simulink model "FFT_32_point_fi_RTL_Implementation"  (R2021a)
settings: Solver=VariableStepAuto  StartTime=0.0  StopTime=0.00001  RelTol=1e-3
undefined symbols (not defined in the file): Input, W16, W2, W32, W4, W8
settings Model: Creator=bahyy  LastModifiedBy=bahyy

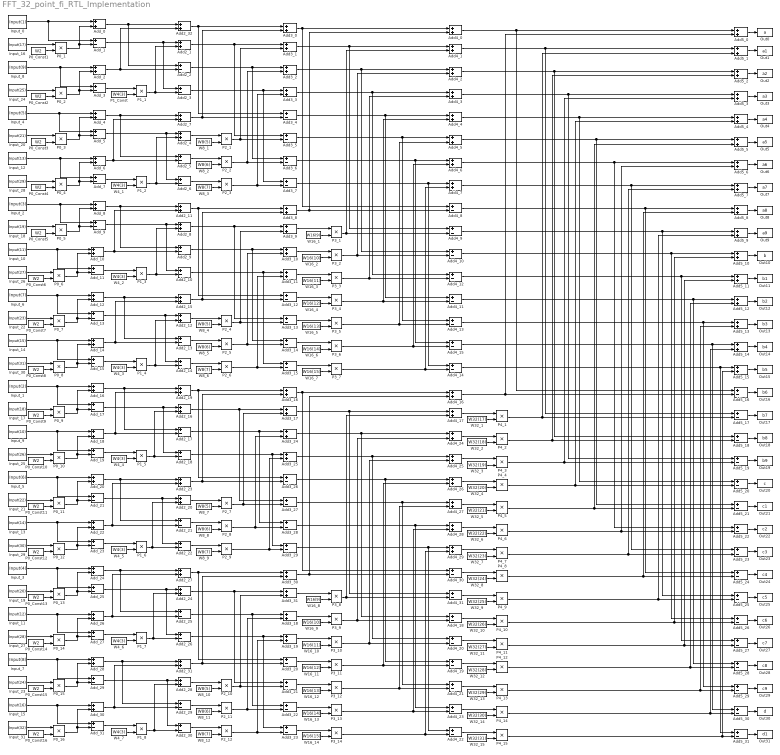
== system FFT_32_point_fi_RTL_Implementation ==
  Add2_{1,4,8,12,16,20,24,28} (8 alike) : Sum  InputSameDT=on  AccumDataTypeStr=fixdt(1,N_bits,W_bits-1)  OutDataTypeStr=fixdt(1,N_bits,W_bits-1)
  Add2_{2..3,5..6,9..10,13..14,17..18,21..22,25..26,29..30} (16 alike) : Sum  Inputs=+-  AccumDataTypeStr=fixdt(1,N_bits,W_bits-1)  OutDataTypeStr=fixdt(1,N_bits,W_bits-1)
  Add2_{7,11,15,19,23,27,31..32} (8 alike) : Sum  AccumDataTypeStr=fixdt(1,N_bits,W_bits-1)  OutDataTypeStr=fixdt(1,N_bits,W_bits-1)
  Add3_{0..3,8..11,16..19,24..25,30..31} (16 alike) : Sum  AccumDataTypeStr=fixdt(1,N_bits,W_bits-1)  OutDataTypeStr=fixdt(1,N_bits,W_bits-1)
  Add3_{4..7,12..15,20..23,26..29} (16 alike) : Sum  Inputs=+-  AccumDataTypeStr=fixdt(1,N_bits,W_bits-1)  OutDataTypeStr=fixdt(1,N_bits,W_bits-1)
  Add4_{0..7,16..17,24..29} (16 alike) : Sum  AccumDataTypeStr=fixdt(1,N_bits,W_bits-1)  OutDataTypeStr=fixdt(1,N_bits,W_bits-1)
  Add4_{8..15,18..23,30..31} (16 alike) : Sum  Inputs=+-  AccumDataTypeStr=fixdt(1,N_bits,W_bits-1)  OutDataTypeStr=fixdt(1,N_bits,W_bits-1)
  Add5_{0..15} (16 alike) : Sum  AccumDataTypeStr=fixdt(1,N_bits,W_bits-1)  OutDataTypeStr=fixdt(1,N_bits,W_bits-1)
  Add5_{16..31} (16 alike) : Sum  Inputs=+-  AccumDataTypeStr=fixdt(1,N_bits,W_bits-1)  OutDataTypeStr=fixdt(1,N_bits,W_bits-1)
  Add_{0,2,4,6,8,10,12,14,16,18,20,22,24,26,28,30} (16 alike) : Sum  AccumDataTypeStr=fixdt(1,N_bits,W_bits-1)  OutDataTypeStr=fixdt(1,N_bits,W_bits-1)
  Add_{1,3,5,7,9,11,13,15,17,19,21,23,25,27,29,31} (16 alike) : Sum  Inputs=+-  AccumDataTypeStr=fixdt(1,N_bits,W_bits-1)  OutDataTypeStr=fixdt(1,N_bits,W_bits-1)
  Input_0 : Constant  Value=Input(1)
  Input_1 : Constant  Value=Input(2)
  Input_10 : Constant  Value=Input(11)
  Input_11 : Constant  Value=Input(12)
  Input_12 : Constant  Value=Input(13)
  Input_13 : Constant  Value=Input(14)
  Input_14 : Constant  Value=Input(15)
  Input_15 : Constant  Value=Input(16)
  Input_16 : Constant  Value=Input(17)
  Input_17 : Constant  Value=Input(18)
  Input_18 : Constant  Value=Input(19)
  Input_19 : Constant  Value=Input(20)
  Input_2 : Constant  Value=Input(3)
  Input_20 : Constant  Value=Input(21)
  Input_21 : Constant  Value=Input(22)
  Input_22 : Constant  Value=Input(23)
  Input_23 : Constant  Value=Input(24)
  Input_24 : Constant  Value=Input(25)
  Input_25 : Constant  Value=Input(26)
  Input_26 : Constant  Value=Input(27)
  Input_27 : Constant  Value=Input(28)
  Input_28 : Constant  Value=Input(29)
  Input_29 : Constant  Value=Input(30)
  Input_3 : Constant  Value=Input(4)
  Input_30 : Constant  Value=Input(31)
  Input_31 : Constant  Value=Input(32)
  Input_4 : Constant  Value=Input(5)
  Input_5 : Constant  Value=Input(6)
  Input_6 : Constant  Value=Input(7)
  Input_7 : Constant  Value=Input(8)
  Input_8 : Constant  Value=Input(9)
  Input_9 : Constant  Value=Input(10)
  Out0 : ToWorkspace  VariableName=a  SampleTime=1
      settings: MaxDataPoints=1  Save2DSignal=2-D array (concatenate along first dimension)
  Out1 : ToWorkspace  VariableName=a1  SampleTime=1
      settings: MaxDataPoints=1  Save2DSignal=2-D array (concatenate along first dimension)
  Out10 : ToWorkspace  VariableName=b  SampleTime=1
      settings: MaxDataPoints=1  Save2DSignal=2-D array (concatenate along first dimension)
  Out11 : ToWorkspace  VariableName=b1  SampleTime=1
      settings: MaxDataPoints=1  Save2DSignal=2-D array (concatenate along first dimension)
  Out12 : ToWorkspace  VariableName=b2  SampleTime=1
      settings: MaxDataPoints=1  Save2DSignal=2-D array (concatenate along first dimension)
  Out13 : ToWorkspace  VariableName=b3  SampleTime=1
      settings: MaxDataPoints=1  Save2DSignal=2-D array (concatenate along first dimension)
  Out14 : ToWorkspace  VariableName=b4  SampleTime=1
      settings: MaxDataPoints=1  Save2DSignal=2-D array (concatenate along first dimension)
  Out15 : ToWorkspace  VariableName=b5  SampleTime=1
      settings: MaxDataPoints=1  Save2DSignal=2-D array (concatenate along first dimension)
  Out16 : ToWorkspace  VariableName=b6  SampleTime=1
      settings: MaxDataPoints=1  Save2DSignal=2-D array (concatenate along first dimension)
  Out17 : ToWorkspace  VariableName=b7  SampleTime=1
      settings: MaxDataPoints=1  Save2DSignal=2-D array (concatenate along first dimension)
  Out18 : ToWorkspace  VariableName=b8  SampleTime=1
      settings: MaxDataPoints=1  Save2DSignal=2-D array (concatenate along first dimension)
  Out19 : ToWorkspace  VariableName=b9  SampleTime=1
      settings: MaxDataPoints=1  Save2DSignal=2-D array (concatenate along first dimension)
  Out2 : ToWorkspace  VariableName=a2  SampleTime=1
      settings: MaxDataPoints=1  Save2DSignal=2-D array (concatenate along first dimension)
  Out20 : ToWorkspace  VariableName=c  SampleTime=1
      settings: MaxDataPoints=1  Save2DSignal=2-D array (concatenate along first dimension)
  Out21 : ToWorkspace  VariableName=c1  SampleTime=1
      settings: MaxDataPoints=1  Save2DSignal=2-D array (concatenate along first dimension)
  Out22 : ToWorkspace  VariableName=c2  SampleTime=1
      settings: MaxDataPoints=1  Save2DSignal=2-D array (concatenate along first dimension)
  Out23 : ToWorkspace  VariableName=c3  SampleTime=1
      settings: MaxDataPoints=1  Save2DSignal=2-D array (concatenate along first dimension)
  Out24 : ToWorkspace  VariableName=c4  SampleTime=1
      settings: MaxDataPoints=1  Save2DSignal=2-D array (concatenate along first dimension)
  Out25 : ToWorkspace  VariableName=c5  SampleTime=1
      settings: MaxDataPoints=1  Save2DSignal=2-D array (concatenate along first dimension)
  Out26 : ToWorkspace  VariableName=c6  SampleTime=1
      settings: MaxDataPoints=1  Save2DSignal=2-D array (concatenate along first dimension)
  Out27 : ToWorkspace  VariableName=c7  SampleTime=1
      settings: MaxDataPoints=1  Save2DSignal=2-D array (concatenate along first dimension)
  Out28 : ToWorkspace  VariableName=c8  SampleTime=1
      settings: MaxDataPoints=1  Save2DSignal=2-D array (concatenate along first dimension)
  Out29 : ToWorkspace  VariableName=c9  SampleTime=1
      settings: MaxDataPoints=1  Save2DSignal=2-D array (concatenate along first dimension)
  Out3 : ToWorkspace  VariableName=a3  SampleTime=1
      settings: MaxDataPoints=1  Save2DSignal=2-D array (concatenate along first dimension)
  Out30 : ToWorkspace  VariableName=d  SampleTime=1
      settings: MaxDataPoints=1  Save2DSignal=2-D array (concatenate along first dimension)
  Out31 : ToWorkspace  VariableName=d1  SampleTime=1
      settings: MaxDataPoints=1  Save2DSignal=2-D array (concatenate along first dimension)
  Out4 : ToWorkspace  VariableName=a4  SampleTime=1
      settings: MaxDataPoints=1  Save2DSignal=2-D array (concatenate along first dimension)
  Out5 : ToWorkspace  VariableName=a5  SampleTime=1
      settings: MaxDataPoints=1  Save2DSignal=2-D array (concatenate along first dimension)
  Out6 : ToWorkspace  VariableName=a6  SampleTime=1
      settings: MaxDataPoints=1  Save2DSignal=2-D array (concatenate along first dimension)
  Out7 : ToWorkspace  VariableName=a7  SampleTime=1
      settings: MaxDataPoints=1  Save2DSignal=2-D array (concatenate along first dimension)
  Out8 : ToWorkspace  VariableName=a8  SampleTime=1
      settings: MaxDataPoints=1  Save2DSignal=2-D array (concatenate along first dimension)
  Out9 : ToWorkspace  VariableName=a9  SampleTime=1
      settings: MaxDataPoints=1  Save2DSignal=2-D array (concatenate along first dimension)
  P0_{1..16} (16 alike) : Product  OutDataTypeStr=fixdt(1,N_bits,W_bits-1)
  P0_Const{1..16} (16 alike) : Constant  Value=W2
  P1_{1..8} (8 alike) : Product  OutDataTypeStr=fixdt(1,N_bits,W_bits-1)
  P1_Const : Constant  Value=W4(3)
  P2_{1..12} (12 alike) : Product  OutDataTypeStr=fixdt(1,N_bits,W_bits-1)
  P3_{1..14} (14 alike) : Product  OutDataTypeStr=fixdt(1,N_bits,W_bits-1)
  P4_{1..15} (15 alike) : Product  OutDataTypeStr=fixdt(1,N_bits,W_bits-1)
  W16_1 : Constant  Value=W16(9)
  W16_10 : Constant  Value=W16(11)
  W16_11 : Constant  Value=W16(12)
  W16_12 : Constant  Value=W16(13)
  W16_13 : Constant  Value=W16(14)
  W16_14 : Constant  Value=W16(15)
  W16_2 : Constant  Value=W16(10)
  W16_3 : Constant  Value=W16(11)
  W16_4 : Constant  Value=W16(12)
  W16_5 : Constant  Value=W16(13)
  W16_6 : Constant  Value=W16(14)
  W16_7 : Constant  Value=W16(15)
  W16_8 : Constant  Value=W16(9)
  W16_9 : Constant  Value=W16(10)
  W32_1 : Constant  Value=W32(17)
  W32_10 : Constant  Value=W32(26)
  W32_11 : Constant  Value=W32(27)
  W32_12 : Constant  Value=W32(28)
  W32_13 : Constant  Value=W32(29)
  W32_14 : Constant  Value=W32(30)
  W32_15 : Constant  Value=W32(31)
  W32_2 : Constant  Value=W32(18)
  W32_3 : Constant  Value=W32(19)
  W32_4 : Constant  Value=W32(20)
  W32_5 : Constant  Value=W32(21)
  W32_6 : Constant  Value=W32(22)
  W32_7 : Constant  Value=W32(23)
  W32_8 : Constant  Value=W32(24)
  W32_9 : Constant  Value=W32(25)
  W4_{1..7} (7 alike) : Constant  Value=W4(3)
  W8_{1,4,7,10} (4 alike) : Constant  Value=W8(5)
  W8_{2,5,8,11} (4 alike) : Constant  Value=W8(6)
  W8_{3,6,9,12} (4 alike) : Constant  Value=W8(7)
  wires:
  Add5_0/1 -> Out0/1
  Add5_6/1 -> Out6/1
  P2_5/1 -> Add3_14/2, Add3_10/2
  Input_4/1 -> Add_5/1, Add_4/1
  P2_1/1 -> Add3_1/2, Add3_5/2
  Add3_6/1 -> Add4_15/1, Add4_6/1
  P3_10/1 -> Add4_20/2, Add4_25/2
  Add5_18/1 -> Out18/1
  W4_1/1 -> P1_2/2
  Add_28/1 -> Add2_29/1, Add2_31/1
  Add2_23/1 -> Add3_26/2, Add3_16/2
  Add5_20/1 -> Out20/1
  Add3_3/1 -> Add4_12/1, Add4_3/1
  Add_14/1 -> Add2_15/2, Add2_13/2
  Add4_17/1 -> P4_1/1
  Add4_13/1 -> Add5_29/1, Add5_13/1
  P4_12/1 -> Add5_28/2, Add5_12/2
  Add_16/1 -> Add2_19/1, Add2_17/1
  P2_11/1 -> Add3_18/2, Add3_22/2
  Add4_7/1 -> Add5_23/1, Add5_7/1
  P2_8/1 -> Add3_28/2, Add3_24/2
  P3_9/1 -> Add4_18/2, Add4_24/2
  W16_6/1 -> P3_6/2
  Add_17/1 -> Add2_18/1, Add2_16/1
  Add4_11/1 -> Add5_28/1, Add5_12/1
  P4_8/1 -> Add5_24/2, Add5_8/2
  W16_4/1 -> P3_4/2
  Add3_11/1 -> P3_3/1
  P4_15/1 -> Add5_31/2, Add5_15/2
  Add5_22/1 -> Out22/1
  Add_23/1 -> P1_6/1
  W16_7/1 -> P3_7/2
  W16_12/1 -> P3_12/2
  Add4_2/1 -> Add5_18/1, Add5_2/1
  Add_31/1 -> P1_8/1
  W32_4/1 -> P4_4/2
  Add_27/1 -> P1_7/1
  P3_4/1 -> Add4_11/2, Add4_4/2
  W16_1/1 -> P3_1/2
  P1_7/1 -> Add2_24/2, Add2_26/2
  W8_5/1 -> P2_5/2
  Add_10/1 -> Add2_11/2, Add2_9/2
  W4_4/1 -> P1_5/2
  Add5_23/1 -> Out23/1
  P3_5/1 -> Add4_13/2, Add4_5/2
  Add_3/1 -> P1_1/1
  P4_5/1 -> Add5_21/2, Add5_5/2
  P1_Const/1 -> P1_1/2
  W32_14/1 -> P4_14/2
  Add5_11/1 -> Out11/1
  Add3_20/1 -> P3_11/1
  Add3_1/1 -> Add4_9/1, Add4_1/1
  Add3_0/1 -> Add4_8/1, Add4_0/1
  Add2_4/1 -> P2_1/1
  Add_24/1 -> Add2_25/1, Add2_27/1
  Add3_30/1 -> Add4_16/2, Add4_30/2
  W4_3/1 -> P1_4/2
  Add_4/1 -> Add2_7/1, Add2_5/1
  Add5_1/1 -> Out1/1
  Add2_8/1 -> Add3_13/1, Add3_9/1
  P4_9/1 -> Add5_25/2, Add5_9/2
  W16_2/1 -> P3_2/2
  P1_4/1 -> Add2_14/2, Add2_12/2
  Add_8/1 -> Add2_9/1, Add2_11/1
  Add5_14/1 -> Out14/1
  Add3_19/1 -> P3_10/1
  Add_9/1 -> Add2_10/1, Add2_8/1
  Add2_1/1 -> Add3_5/1, Add3_1/1
  Add_6/1 -> Add2_7/2, Add2_5/2
  Add4_4/1 -> Add5_20/1, Add5_4/1
  Add_1/1 -> Add2_3/1, Add2_1/1
  Add2_10/1 -> Add3_15/1, Add3_11/1
  W4_2/1 -> P1_3/2
  Add2_27/1 -> Add3_20/1, Add3_30/1
  W32_9/1 -> P4_9/2
  Add5_27/1 -> Out27/1
  W16_14/1 -> P3_14/2
  Add5_3/1 -> Out3/1
  Add5_15/1 -> Out15/1
  P2_2/1 -> Add3_6/2, Add3_2/2
  W4_7/1 -> P1_8/2
  Add_30/1 -> Add2_29/2, Add2_31/2
  P4_7/1 -> Add5_23/2, Add5_7/2
  P1_8/1 -> Add2_30/2, Add2_28/2
  P3_7/1 -> Add4_14/2, Add4_7/2
  P4_1/1 -> Add5_17/2, Add5_1/2
  W16_9/1 -> P3_9/2
  Add4_26/1 -> P4_4/1
  W32_1/1 -> P4_1/2
  Add_2/1 -> Add2_32/2, Add2_2/2
  Add_0/1 -> Add2_32/1, Add2_2/1
  Add5_26/1 -> Out26/1
  P2_7/1 -> Add3_17/2, Add3_27/2
  Add5_29/1 -> Out29/1
  P3_8/1 -> Add4_17/2, Add4_31/2
  Add_25/1 -> Add2_24/1, Add2_26/1
  Add2_22/1 -> P2_9/1
  Add3_16/1 -> Add4_16/1, Add4_30/1
  P3_12/1 -> Add4_27/2, Add4_21/2
  Add2_17/1 -> Add3_28/1, Add3_24/1
  P1_6/1 -> Add2_22/2, Add2_20/2
  W8_7/1 -> P2_7/2
  P4_3/1 -> Add5_19/2, Add5_3/2
  W8_2/1 -> P2_2/2
  Add4_1/1 -> Add5_1/1, Add5_17/1
  W32_3/1 -> P4_3/2
  Add2_25/1 -> Add3_18/1, Add3_22/1
  Add5_19/1 -> Out19/1
  Add2_19/1 -> Add3_26/1, Add3_16/1
  Add5_21/1 -> Out21/1
  P3_13/1 -> Add4_28/2, Add4_23/2
  Add2_3/1 -> Add3_7/1, Add3_3/1
  Add2_26/1 -> Add3_19/1, Add3_23/1
  Add4_21/1 -> P4_13/1
  P1_1/1 -> Add2_3/2, Add2_1/2
  P3_3/1 -> Add4_12/2, Add4_3/2
  Add5_5/1 -> Out5/1
  W32_10/1 -> P4_10/2
  W8_10/1 -> P2_10/2
  W16_13/1 -> P3_13/2
  P3_6/1 -> Add4_15/2, Add4_6/2
  W4_6/1 -> P1_7/2
  Add_5/1 -> Add2_6/1, Add2_4/1
  P4_6/1 -> Add5_22/2, Add5_6/2
  Add5_16/1 -> Out16/1
  Add2_16/1 -> Add3_17/1, Add3_27/1
  Add5_30/1 -> Out30/1
  W16_5/1 -> P3_5/2
  Add_19/1 -> P1_5/1
  W32_12/1 -> P4_12/2
  W8_1/1 -> P2_1/2
  W32_7/1 -> P4_7/2
  Add4_31/1 -> P4_9/1
  P4_11/1 -> Add5_27/2, Add5_11/2
  Add2_20/1 -> P2_7/1
  W32_11/1 -> P4_11/2
  W8_12/1 -> P2_12/2
  W32_5/1 -> P4_5/2
  Add4_22/1 -> P4_15/1
  Add4_3/1 -> Add5_19/1, Add5_3/1
  Add4_18/1 -> P4_10/1
  Add3_21/1 -> P3_12/1
  Add_18/1 -> Add2_19/2, Add2_17/2
  Add2_5/1 -> P2_2/1
  Add2_7/1 -> Add3_0/2, Add3_4/2
  P4_13/1 -> Add5_29/2, Add5_13/2
  Add5_9/1 -> Out9/1
  Add4_5/1 -> Add5_21/1, Add5_5/1
  P2_10/1 -> Add3_31/2, Add3_21/2
  Add4_28/1 -> P4_6/1
  Input_8/1 -> Add_3/1, Add_2/1
  Add4_0/1 -> Add5_0/1, Add5_16/1
  W32_13/1 -> P4_13/2
  Add5_13/1 -> Out13/1
  Add2_24/1 -> Add3_31/1, Add3_21/1
  Add_11/1 -> P1_3/1
  P3_11/1 -> Add4_19/2, Add4_26/2
  Add5_2/1 -> Out2/1
  Add4_29/1 -> P4_7/1
  Add2_30/1 -> P2_12/1
  Add_22/1 -> Add2_21/2, Add2_23/2
  Add3_29/1 -> Add4_29/1, Add4_22/1
  Add2_14/1 -> P2_6/1
  Add_20/1 -> Add2_21/1, Add2_23/1
  Add5_10/1 -> Out10/1
  Add3_22/1 -> P3_13/1
  P2_3/1 -> Add3_7/2, Add3_3/2
  W8_4/1 -> P2_4/2
  Add3_23/1 -> P3_14/1
  Add2_31/1 -> Add3_20/2, Add3_30/2
  Add2_12/1 -> P2_4/1
  W32_2/1 -> P4_2/2
  Add3_7/1 -> Add4_14/1, Add4_7/1
  P3_14/1 -> Add4_29/2, Add4_22/2
  Add4_20/1 -> P4_11/1
  Add3_18/1 -> P3_9/1
  Add4_30/1 -> P4_8/1
  Add4_23/1 -> P4_14/1
  Add4_16/1 -> Add5_16/2, Add5_0/2
  P4_2/1 -> Add5_18/2, Add5_2/2
  Add3_26/1 -> Add4_19/1, Add4_26/1
  Add2_28/1 -> P2_10/1
  Add4_27/1 -> P4_5/1
  W8_3/1 -> P2_3/2
  Add4_14/1 -> Add5_31/1, Add5_15/1
  W16_8/1 -> P3_8/2
  P4_10/1 -> Add5_26/2, Add5_10/2
  Add_12/1 -> Add2_15/1, Add2_13/1
  Add4_9/1 -> Add5_25/1, Add5_9/1
  P2_9/1 -> Add3_29/2, Add3_25/2
  Add3_5/1 -> Add4_13/1, Add4_5/1
  W16_3/1 -> P3_3/2
  Add2_2/1 -> Add3_6/1, Add3_2/1
  Add2_21/1 -> P2_8/1
  Add2_18/1 -> Add3_29/1, Add3_25/1
  Add2_29/1 -> P2_11/1
  Add3_31/1 -> P3_8/1
  Add4_19/1 -> P4_12/1
  P1_3/1 -> Add2_10/2, Add2_8/2
  P2_6/1 -> Add3_15/2, Add3_11/2
  Add3_10/1 -> P3_2/1
  Add5_28/1 -> Out28/1
  Add5_12/1 -> Out12/1
  Add4_6/1 -> Add5_22/1, Add5_6/1
  W32_8/1 -> P4_8/2
  Add_15/1 -> P1_4/1
  Add3_25/1 -> Add4_20/1, Add4_25/1
  W32_15/1 -> P4_15/2
  Add5_8/1 -> Out8/1
  Add2_15/1 -> Add3_12/2, Add3_8/2
  Add5_31/1 -> Out31/1
  Add3_27/1 -> Add4_27/1, Add4_21/1
  P4_14/1 -> Add5_30/2, Add5_14/2
  P1_5/1 -> Add2_18/2, Add2_16/2
  Add5_25/1 -> Out25/1
  P3_2/1 -> Add4_10/2, Add4_2/2
  W8_6/1 -> P2_6/2
  Add3_24/1 -> Add4_18/1, Add4_24/1
  Add_21/1 -> Add2_22/1, Add2_20/1
  Add5_17/1 -> Out17/1
  Add3_9/1 -> P3_1/1
  Add4_25/1 -> P4_3/1
  P1_2/1 -> Add2_6/2, Add2_4/2
  P2_4/1 -> Add3_13/2, Add3_9/2
  Add5_24/1 -> Out24/1
  Add_29/1 -> Add2_30/1, Add2_28/1
  W32_6/1 -> P4_6/2
  W16_10/1 -> P3_10/2
  Add4_12/1 -> Add5_27/1, Add5_11/1
  W16_11/1 -> P3_11/2
  W8_8/1 -> P2_8/2
  Add3_13/1 -> P3_5/1
  P2_12/1 -> Add3_19/2, Add3_23/2
  Add_26/1 -> Add2_25/2, Add2_27/2
  Add3_2/1 -> Add4_10/1, Add4_2/1
  Add3_12/1 -> P3_4/1
  Add3_17/1 -> Add4_17/1, Add4_31/1
  Add4_24/1 -> P4_2/1
  Add3_15/1 -> P3_7/1
  Add2_13/1 -> P2_5/1
  Add3_28/1 -> Add4_28/1, Add4_23/1
  Add_13/1 -> Add2_14/1, Add2_12/1
  Add3_14/1 -> P3_6/1
  W8_9/1 -> P2_9/2
  W8_11/1 -> P2_11/2
  Add2_6/1 -> P2_3/1
  Add2_11/1 -> Add3_12/1, Add3_8/1
  Input_12/1 -> Add_7/1, Add_6/1
  P3_1/1 -> Add4_9/2, Add4_1/2
  P4_4/1 -> Add5_20/2, Add5_4/2
  Input_0/1 -> Add_1/1, Add_0/1
  Add3_8/1 -> Add4_0/2, Add4_8/2
  Add2_9/1 -> Add3_14/1, Add3_10/1
  Add4_8/1 -> Add5_24/1, Add5_8/1
  Add3_4/1 -> Add4_11/1, Add4_4/1
  Add2_32/1 -> Add3_4/1, Add3_0/1
  Add5_7/1 -> Out7/1
  Add4_15/1 -> Add5_30/1, Add5_14/1
  Add5_4/1 -> Out4/1
  W4_5/1 -> P1_6/2
  Add_7/1 -> P1_2/1
  Add4_10/1 -> Add5_26/1, Add5_10/1
  P0_Const1/1 -> P0_1/2
  Input_16/1 -> P0_1/1
  P0_1/1 -> Add_1/2, Add_0/2
  P0_Const2/1 -> P0_2/2
  Input_24/1 -> P0_2/1
  P0_2/1 -> Add_3/2, Add_2/2
  P0_Const3/1 -> P0_3/2
  Input_20/1 -> P0_3/1
  P0_3/1 -> Add_5/2, Add_4/2
  P0_Const4/1 -> P0_4/2
  Input_28/1 -> P0_4/1
  P0_4/1 -> Add_7/2, Add_6/2
  Input_18/1 -> P0_5/1
  P0_5/1 -> Add_9/2, Add_8/2
  P0_Const5/1 -> P0_5/2
  Input_2/1 -> Add_9/1, Add_8/1
  Input_26/1 -> P0_6/1
  P0_6/1 -> Add_11/2, Add_10/2
  P0_Const6/1 -> P0_6/2
  Input_10/1 -> Add_11/1, Add_10/1
  Input_22/1 -> P0_7/1
  P0_7/1 -> Add_13/2, Add_12/2
  P0_Const7/1 -> P0_7/2
  Input_6/1 -> Add_13/1, Add_12/1
  Input_30/1 -> P0_8/1
  P0_8/1 -> Add_15/2, Add_14/2
  P0_Const8/1 -> P0_8/2
  Input_14/1 -> Add_15/1, Add_14/1
  Input_17/1 -> P0_9/1
  P0_9/1 -> Add_17/2, Add_16/2
  P0_Const9/1 -> P0_9/2
  Input_1/1 -> Add_17/1, Add_16/1
  Input_25/1 -> P0_10/1
  P0_10/1 -> Add_19/2, Add_18/2
  P0_Const10/1 -> P0_10/2
  Input_9/1 -> Add_19/1, Add_18/1
  Input_21/1 -> P0_11/1
  P0_11/1 -> Add_21/2, Add_20/2
  P0_Const11/1 -> P0_11/2
  Input_5/1 -> Add_21/1, Add_20/1
  Input_29/1 -> P0_12/1
  P0_12/1 -> Add_23/2, Add_22/2
  P0_Const12/1 -> P0_12/2
  Input_13/1 -> Add_23/1, Add_22/1
  Input_19/1 -> P0_13/1
  P0_13/1 -> Add_25/2, Add_24/2
  P0_Const13/1 -> P0_13/2
  Input_3/1 -> Add_25/1, Add_24/1
  Input_27/1 -> P0_14/1
  P0_14/1 -> Add_27/2, Add_26/2
  P0_Const14/1 -> P0_14/2
  Input_11/1 -> Add_27/1, Add_26/1
  Input_23/1 -> P0_15/1
  P0_15/1 -> Add_29/2, Add_28/2
  P0_Const15/1 -> P0_15/2
  Input_7/1 -> Add_29/1, Add_28/1
  Input_31/1 -> P0_16/1
  P0_16/1 -> Add_31/2, Add_30/2
  P0_Const16/1 -> P0_16/2
  Input_15/1 -> Add_31/1, Add_30/1
